simulink model "vexarmcortex_BEST_IR_Sensor_LineFollower3"  (R2019a)
settings: Solver=FixedStepAuto  StartTime=0.0  StopTime=inf  RelTol=1e-3
libraries: vexarmcortexlib x5
settings Model: ExtModeTrigDuration=25  Creator=The MathWorks, Inc.  LastModifiedBy=josea
settings DataIOCC: ReturnWorkspaceOutputs=off
settings OptimizationCC: MaxStackSize=64
settings DebuggingCC: ParameterTunabilityLossMsg=error  ArithmeticOperatorsInVariantConditions=warning
settings HardwareCC: ProdBitPerPointer=32  ProdBitPerSizeT=32  ProdBitPerPtrDiffT=32  ProdLargestAtomicInteger=Long  ProdLargestAtomicFloat=Double  ProdWordSize=32  ProdHWDeviceType=ARM Compatible->ARM Cortex  UseEmbeddedCoderFeatures=off
settings SFSimCC: SimUseLocalCustomCode=off
settings RTWCC: SystemTargetFile=ert.tlc  HardwareBoard=ARM Cortex-based VEX Microcontroller  TLCOptions="-aInlineSetEventsForThisBaseRateFcn=TLC_FALSE -aSuppressMultiTaskScheduler=TLC_FALSE  -aRateBasedStepFcn=0"  TemplateMakefile=ert_default_tmf  GenerateReport=on  RTWUseLocalCustomCode=off  Toolchain=GNU Tools for VEX ARM Cortex  LaunchReport=on
settings CodeAppCC: ForceParamTrailComments=on  OperatorAnnotations=on  StateflowObjectComments=on  MATLABSourceComments=on
settings ERTTargetCC: ERTCustomFileBanners=off  SupportContinuousTime=on  SupportNonInlinedSFcns=on  RemoveResetFunc=off  ModelStepFunctionPrototypeControlCompliant=off

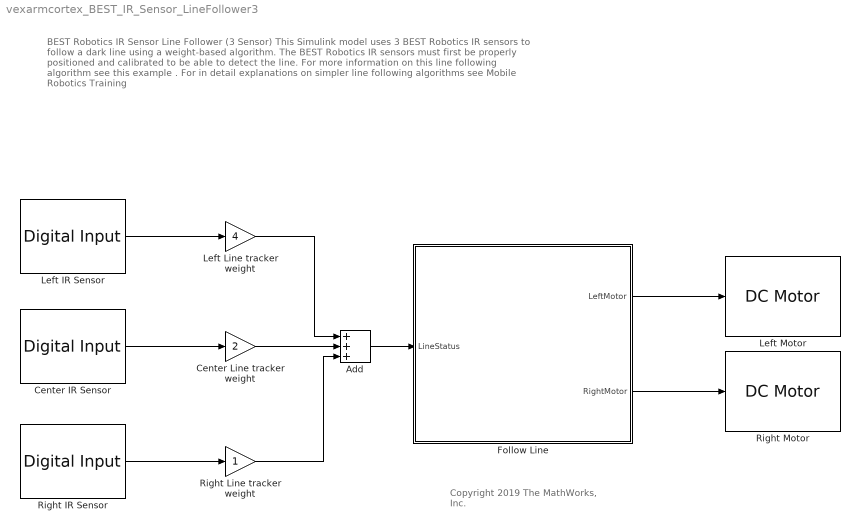
== system vexarmcortex_BEST_IR_Sensor_LineFollower3 ==
  note: BEST Robotics IR Sensor Line Follower (3 Sensor)
      |
      | This Simulink model uses 3 BEST Robotics IR sensors to follow a dark line using a weight-based algorithm.
      | The BEST Robotics IR sensors must first be properly positioned and calibrated to be able to detect the line.
      | For more information on this line following algorithm see this example .
      | For in detail explanations on simpler line following algorithms see Mobile Robotics Training
  note: Copyright 2019 The MathWorks, Inc.
  Add : Sum  Inputs=+++
  Center IR Sensor : vexarmcortexlib/Sensors/Digital Input  inChan=4  SimulationIn=off  SampleTime=0.05
      settings: SourceProductName=Simulink Coder Support Package for ARM Cortex-based VEX Microcontroller  SourceProductBaseCode=EC_VEX_MICRO
  Center Line tracker weight : Gain  Gain=2
  Follow Line : Stateflow chart  TreatAsAtomicUnit=on
  Left IR Sensor : vexarmcortexlib/Sensors/Digital Input  inChan=4  SimulationIn=off  SampleTime=0.05
      settings: SourceProductName=Simulink Coder Support Package for ARM Cortex-based VEX Microcontroller  SourceProductBaseCode=EC_VEX_MICRO
  Left Line tracker weight : Gain  Gain=4
  Left Motor : vexarmcortexlib/Actuators/DC Motor  motor=4  scaleFactor=1/13.5  SimulationOut=off
      settings: SourceProductName=Simulink Coder Support Package for ARM Cortex-based VEX Microcontroller  SourceProductBaseCode=EC_VEX_MICRO
  Right IR Sensor : vexarmcortexlib/Sensors/Digital Input  inChan=4  SimulationIn=off  SampleTime=0.05
      settings: SourceProductName=Simulink Coder Support Package for ARM Cortex-based VEX Microcontroller  SourceProductBaseCode=EC_VEX_MICRO
  Right Line tracker weight : Gain
  Right Motor : vexarmcortexlib/Actuators/DC Motor  motor=3  scaleFactor=1/13.5  SimulationOut=off
      settings: SourceProductName=Simulink Coder Support Package for ARM Cortex-based VEX Microcontroller  SourceProductBaseCode=EC_VEX_MICRO
  wires:
  Center Line tracker weight/1 -> Add/2
  Left Line tracker weight/1 -> Add/1
  Add/1 -> Follow Line/1(LineStatus)
  Follow Line/1(LeftMotor) -> Left Motor/1
  Follow Line/2(RightMotor) -> Right Motor/1
  Right Line tracker weight/1 -> Add/3
  Left IR Sensor/1 -> Left Line tracker weight/1
  Center IR Sensor/1 -> Center Line tracker weight/1
  Right IR Sensor/1 -> Right Line tracker weight/1

== stateflow chart vexarmcortex_BEST_IR_Sensor_LineFollower3/Follow Line ==
  state Straight
    during:
    LeftMotor=-20;
    RightMotor=20;
  state TurnLeft
    during:
    LeftMotor=30;
    RightMotor=30;
  state TurnRight
    during:
    LeftMotor=-30;
    RightMotor=-30;
  state EndOfLine
    during:
    LeftMotor=0;
    RightMotor=0;
  (default) -> Straight
  Straight -> TurnRight [order 2] : [LineStatus == 1 || LineStatus == 3]
  Straight -> TurnLeft [order 1] : [LineStatus == 4 || LineStatus == 6]
  TurnLeft -> Straight [order 1] : [LineStatus == 0 || LineStatus == 2]
  TurnRight -> Straight [order 1] : [LineStatus == 0 || LineStatus == 2]
  Straight -> EndOfLine [order 3] : [LineStatus == 7]
  EndOfLine -> Straight [order 1] : [LineStatus == 0 || LineStatus == 2]
  TurnRight -> TurnLeft [order 2] : [LineStatus == 4 || LineStatus == 6]
  TurnLeft -> TurnRight [order 2] : [LineStatus == 1 || LineStatus == 3]
  EndOfLine -> TurnLeft [order 3] : [LineStatus == 4 || LineStatus == 6]
  TurnLeft -> EndOfLine [order 3] : [LineStatus == 7]
  TurnRight -> EndOfLine [order 3] : [LineStatus == 7]
  EndOfLine -> TurnRight [order 2] : [LineStatus == 1 || LineStatus == 3]
  data: LineStatus input; LeftMotor output; RightMotor output
